simulink library "PostmixLib"  (R2022b)
settings: Solver=VariableStepAuto  StartTime=0.0  StopTime=10.0  RelTol=1e-3
settings Model: Creator=ak1044356  LastModifiedBy=sa1045272
settings SolverCC: AlgebraicLoopSolver=TrustRegion
settings DebuggingCC: UnconnectedInputMsg=warning  UnconnectedOutputMsg=warning  UnconnectedLineMsg=warning  SFMachineParentedDataDiag=warning  ArithmeticOperatorsInVariantConditions=warning
settings ModelReferenceCC: EnableRefExpFcnMdlSchedulingChecks=on
settings SFSimCC: CustomCodeUndefinedFunction=UseInterfaceOnly

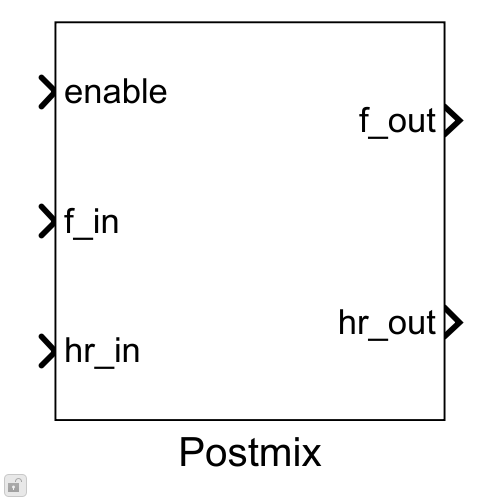
[thumbnail: Simulink's stored preview of the top-level diagram]
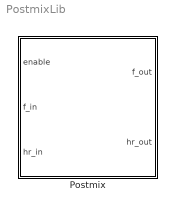
== system PostmixLib ==
  Postmix : Subsystem

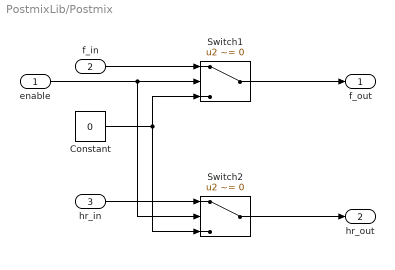
== system PostmixLib/Postmix ==
  enable : Inport
  f_in : Inport  Port=2  OutDataTypeStr=single
  hr_in : Inport  Port=3  OutDataTypeStr=single
  Constant : Constant  Value=0  OutDataTypeStr=single
  Switch1 : Switch  Criteria=u2 ~= 0  Threshold=.5  ZeroCross=off  SaturateOnIntegerOverflow=off  InputSameDT=off
  Switch2 : Switch  Criteria=u2 ~= 0  Threshold=.5  ZeroCross=off  SaturateOnIntegerOverflow=off  InputSameDT=off
  f_out : Outport  VectorParamsAs1DForOutWhenUnconnected=off
  hr_out : Outport  Port=2  VectorParamsAs1DForOutWhenUnconnected=off
  wires:
  f_in/1 -> Switch1/1
  Switch1/1 -> f_out/1
  hr_in/1 -> Switch2/1
  Switch2/1 -> hr_out/1
  Constant/1 -> Switch2/3, Switch1/3
  enable/1 -> Switch2/2, Switch1/2
